simulink model "F16BlockASYM_JOY"  (R2012b)
settings: Solver=ode5  StartTime=0.0  StopTime=inf  FixedStep=0.02  RelTol=1e-3
InitFcn:
  | mex nlplantASYM.c
values from neighbouring files (symbols this model uses):
  DisEle_1 = ElevatorDis    (= 0)    [runF16Sim.m]
  DisEle_2 = -2*ElevatorDis    (= 0)    [runF16Sim.m]
  DisEle_3 = ElevatorDis    (= 0)    [runF16Sim.m]
  fi_flag_Simulink = 1    [runF16Sim.m]
  latitude = 52.073105    [runF16Sim.m]
  longitude = -000.616697    (= -0.616697)    [runF16Sim.m]
  Model_used_flag = 1    [runF16Sim.m]
undefined symbols (not defined in the file or in its folder): Earth, m, rad, s, trim_control, trim_state, trim_throttle, WGS84
libraries: F16_Actuator_Library x7, simulink x7, aerolibfltsims x3, aerolibtransform2 x2, aerolibconvert2 x2, aerolibatmos2 x2, aerolibasang x1, aerolibanimutils x1, aerolibconvert x1, aerolibobsolete x1, vrlib x1
settings Model: ExtModeAutoUpdateStatusClock=off  Creator=keviczky  LastModifiedBy=David
settings DataIOCC: Decimation=50  LimitDataPoints=off  SignalLoggingSaveFormat=ModelDataLogs  SignalLoggingName=sigsOut
settings OptimizationCC: BooleanDataType=off  InlineInvariantSignals=on
settings DebuggingCC: SaveWithParameterizedLinksMsg=none  SignalResolutionControl=TryResolveAllWithWarning  SolverPrmCheckMsg=none  MultiTaskDSMMsg=warning  MultiTaskCondExecSysMsg=none  StrictBusMsg=None
settings HardwareCC: TargetUnknown=on
settings RTWCC: IncludeERTFirstTime=on
settings GRTTargetCC: CombineOutputUpdateFcns=off  GRTInterface=on

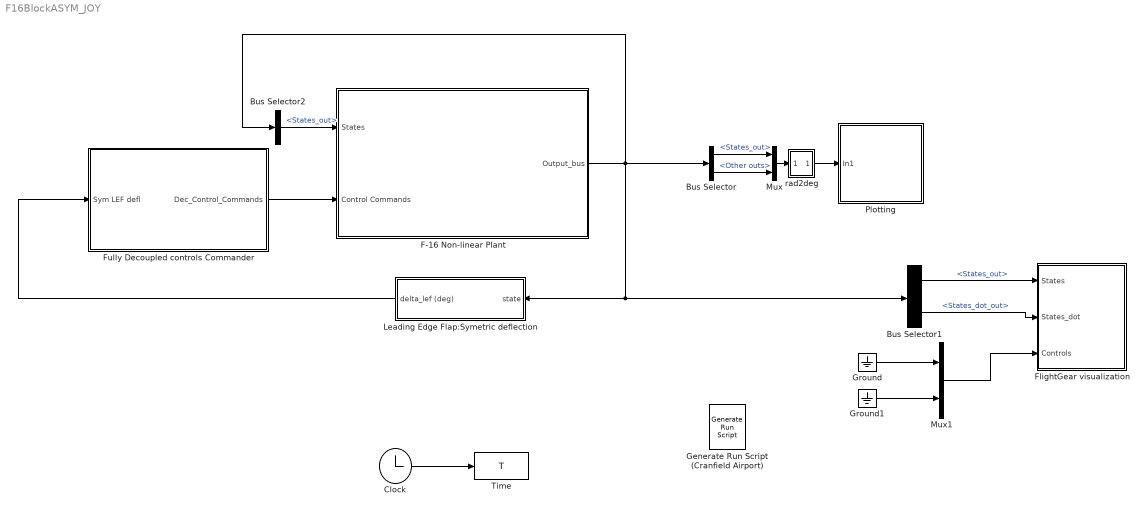
== system F16BlockASYM_JOY ==
  Bus Selector : BusSelector  OutputSignals=States_out,Other outs
  Bus Selector1 : BusSelector  OutputSignals=States_out,States_dot_out
  Bus Selector2 : BusSelector  OutputSignals=States_out
  Clock : Clock
      settings: Decimation=50
  F-16 Non-linear Plant : Subsystem
      mask Display:
      | image(imread('f16.jpg'))
      | port_label('output', 1, 'Out_bus')
      | port_label('input', 1, 'State_feedback')
      | port_label('input', 2, 'Control_Commands')
  FlightGear visualization : Subsystem  TreatAsAtomicUnit=on
  Fully Decoupled controls Commander : Subsystem
  Generate Run Script (Cranfield Airport) : aerolibfltsims/Generate Run Script  OutputFileName=runfg.bat  FlightGearBaseDirectory=C:\Program Files\FlightGear  GeometryModelName=f16  DestinationPort=5502  OriginAddress=127.0.0.1  OriginPort=5505  LocalAddress=127.0.0.1  AirportId=EGTC  RunwayId=1  InitialAltitude=trim_state(3)*3.2808399  InitialHeading=0  OffsetDistance=4.72  OffsetAzimuth=0  GenerateFile=off  Architecture=Win64  dataFlow=Send
  Ground : Ground
  Ground1 : Ground
  Leading Edge Flap:Symetric deflection : Subsystem
  Mux : Mux  Inputs=2
  Mux1 : Mux  Inputs=2
  Plotting : Subsystem
      mask Display: image(imread('f16output.jpg'))
  Time : ToWorkspace  VariableName=T  SampleTime=-1
      settings: Decimation=100
  rad2deg : Subsystem
  wires:
  Fully Decoupled controls Commander/1(Dec_Control_Commands) -> F-16 Non-linear Plant/2(Control Commands)
  Clock/1 -> Time/1
  rad2deg/1(Out1) -> Plotting/1(In1)
  Bus Selector/1 -> Mux/1  "<States_out>"
  Bus Selector/2 -> Mux/2  "<Other outs>"
  Mux/1 -> rad2deg/1(In1)
  F-16 Non-linear Plant/1(Output_bus) -> Bus Selector1/1, Leading Edge Flap:Symetric deflection/1(state), Bus Selector2/1, Bus Selector/1
  Bus Selector2/1 -> F-16 Non-linear Plant/1(States)  "<States_out>"
  Leading Edge Flap:Symetric deflection/1(delta_lef (deg)) -> Fully Decoupled controls Commander/1(Sym LEF defl)
  Ground/1 -> Mux1/1
  Ground1/1 -> Mux1/2
  Bus Selector1/1 -> FlightGear visualization/1(States)  "<States_out>"
  Bus Selector1/2 -> FlightGear visualization/2(States_dot)  "<States_dot_out>"
  Mux1/1 -> FlightGear visualization/3(Controls)

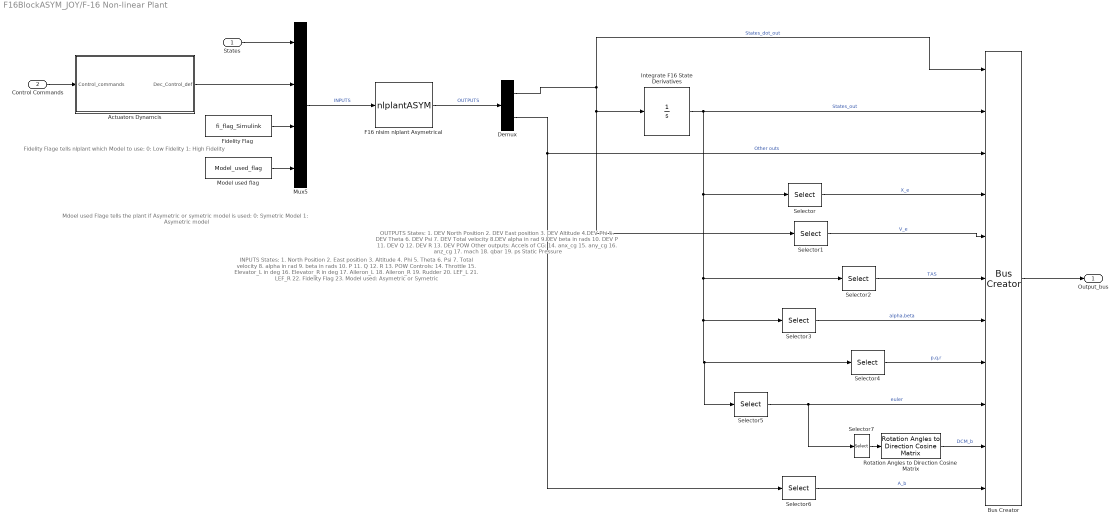
== system F16BlockASYM_JOY/F-16 Non-linear Plant ==
  note: OUTPUTS
      | States:
      | 1. DEV North Position
      | 2. DEV East position
      | 3. DEV Altitude
      | 4.DEV  Phi
      | 5. DEV Theta
      | 6. DEV Psi
      | 7. DEV Total velocity
      | 8.DEV alpha in rad
      | 9.DEV  beta in rads
      | 10. DEV P
      | 11. DEV Q
      | 12. DEV R
      | 13. DEV POW
      |
      | Other outputs:
      | Accels of CG:
      | 14. anx_cg
      | 15. any_cg
      | 16. anz_cg
      | 17. mach
      | 18. qbar
      | 19. ps   Static Pressure
  note: Fidelity Flage tells nlplant
      | which Model to use:
      | 0: Low Fidelity
      | 1: High Fidelity
  note: INPUTS
      | States:
      | 1. North Position
      | 2. East position
      | 3. Altitude
      | 4. Phi
      | 5. Theta
      | 6. Psi
      | 7. Total velocity
      | 8. alpha in rad
      | 9. beta in rads
      | 10. P
      | 11. Q
      | 12. R
      | 13. POW
      |
      | Controls:
      | 14. Throttle
      | 15. Elevator_L in deg
      | 16. Elevator_R in deg
      | 17. Aileron_L
      | 18. Aileron_R
      | 19. Rudder
      | 20. LEF_L
      | 21. LEF_R
      |
      | 22. Fidelity Flag
      |
      | 23. Model used: Asymetric or Symetric
  note: Mdoel used  Flage tells the plant
      |  if Asymetric or symetric model is used:
      | 0: Symetric Model
      | 1: Asymetric model
  States : Inport
  Control Commands : Inport  Port=2
  Actuators Dynamcis : Subsystem  TreatAsAtomicUnit=on
  Bus Creator : BusCreator  Inputs=11
  Demux : Demux  Outputs=[13 6]
  F16 nlsim nlplant Asymetrical : MATLABFcn  MATLABFcn=nlplantASYM  OutputDimensions=19  OutputSignalType=real
  Fidelity Flag : Constant  Value=fi_flag_Simulink
  Integrate F16 State Derivatives : Integrator  InitialCondition=trim_state
  Model used flag : Constant  Value=Model_used_flag
  Mux5 : Mux  Inputs=[13 8 1 1]
  Rotation Angles to Direction Cosine Matrix : aerolibtransform2/Rotation Angles to Direction Cosine Matrix  rotationOrder=ZYX
  Selector : Selector  InputPortWidth=13  IndexOptions=Index vector (dialog)  Indices=[1:3]  OutputSizes=1
  Selector1 : Selector  InputPortWidth=13  IndexOptions=Index vector (dialog)  Indices=[1:3]  OutputSizes=1
  Selector2 : Selector  InputPortWidth=13  IndexOptions=Index vector (dialog)  Indices=[7]  OutputSizes=1
  Selector3 : Selector  InputPortWidth=13  IndexOptions=Index vector (dialog)  Indices=[8:9]  OutputSizes=1
  Selector4 : Selector  InputPortWidth=13  IndexOptions=Index vector (dialog)  Indices=[10:12]  OutputSizes=1
  Selector5 : Selector  InputPortWidth=13  IndexOptions=Index vector (dialog)  Indices=[4:6]  OutputSizes=1
  Selector6 : Selector  InputPortWidth=6  IndexOptions=Index vector (dialog)  Indices=[1:3]  OutputSizes=1
  Selector7 : Selector  InputPortWidth=3  IndexOptions=Index vector (dialog)  Indices=[3 2 1]  OutputSizes=1
  Output_bus : Outport
  wires:
  Demux/1 -> Bus Creator/1, Selector1/1, Integrate F16 State Derivatives/1  "States_dot_out"
  Selector/1 -> Bus Creator/4  "X_e"
  Selector1/1 -> Bus Creator/5  "V_e"
  Selector2/1 -> Bus Creator/6  "TAS"
  Selector3/1 -> Bus Creator/7  "alpha,beta"
  Selector4/1 -> Bus Creator/8  "p,q,r"
  Selector5/1 -> Selector7/1, Bus Creator/9  "euler"
  Selector6/1 -> Bus Creator/11  "A_b"
  Demux/2 -> Selector6/1, Bus Creator/3  "Other outs"
  Selector7/1 -> Rotation Angles to Direction Cosine Matrix/1
  Integrate F16 State Derivatives/1 -> Selector5/1, Selector4/1, Selector3/1, Selector2/1, Selector/1, Bus Creator/2  "States_out"
  Rotation Angles to Direction Cosine Matrix/1 -> Bus Creator/10  "DCM_b"
  Bus Creator/1 -> Output_bus/1
  Fidelity Flag/1 -> Mux5/3
  Control Commands/1 -> Actuators Dynamcis/1(Control_commands)
  States/1 -> Mux5/1
  Mux5/1 -> F16 nlsim nlplant Asymetrical/1  "INPUTS"
  F16 nlsim nlplant Asymetrical/1 -> Demux/1  "OUTPUTS"
  Actuators Dynamcis/1(Dec_Control_def) -> Mux5/2
  Model used flag/1 -> Mux5/4

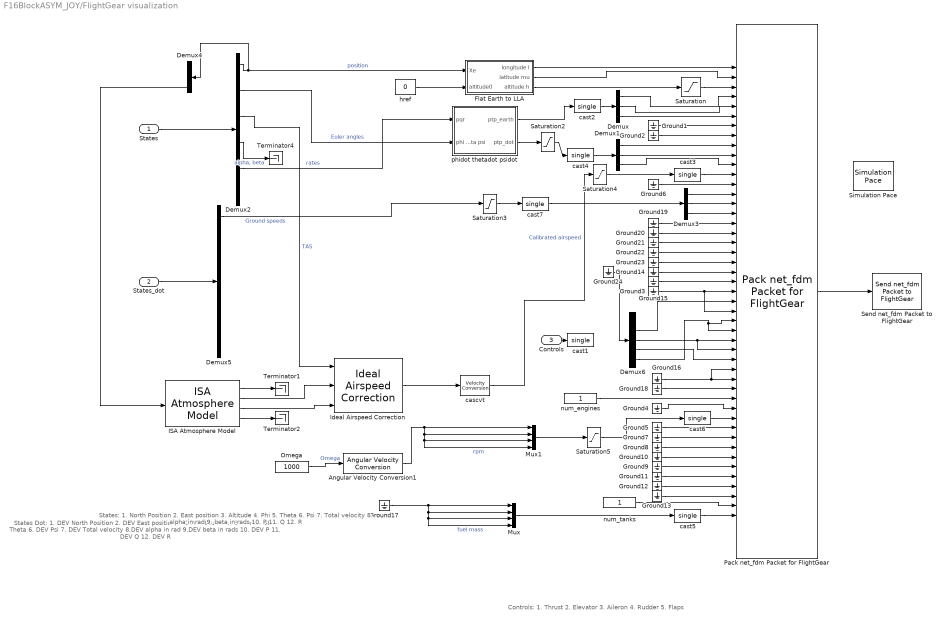
== system F16BlockASYM_JOY/FlightGear visualization ==
  note: States Dot:
      | 1. DEV North Position
      | 2. DEV East position
      | 3. DEV Altitude
      | 4.DEV  Phi
      | 5. DEV Theta
      | 6. DEV Psi
      | 7. DEV Total velocity
      | 8.DEV alpha in rad
      | 9.DEV  beta in rads
      | 10. DEV P
      | 11. DEV Q
      | 12. DEV R
  note: States:
      | 1. North Position
      | 2. East position
      | 3. Altitude
      | 4. Phi
      | 5. Theta
      | 6. Psi
      | 7. Total velocity
      | 8. alpha in rad
      | 9. beta in rads
      | 10. P
      | 11. Q
      | 12. R
  note: Controls:
      | 1. Thrust
      | 2. Elevator
      | 3. Aileron
      | 4. Rudder
      | 5. Flaps
  States : Inport
  States_dot : Inport  Port=2
  Controls : Inport  Port=3
  Angular Velocity Conversion1 : aerolibconvert2/Angular Velocity Conversion  IU=rad/s  OU=rpm
  Demux{,1,3..4} (4 alike) : Demux  Outputs=3
  Demux2 : Demux  Outputs=[3 3 1 2 3 1]
  Demux5 : Demux  Outputs=[3 3 1 2 3 1]
  Demux6 : Demux  Outputs=5
  Flat Earth to LLA : Subsystem
  Ground{1..24} (24 alike) : Ground
  ISA Atmosphere Model : aerolibatmos2/ISA Atmosphere Model  custom=off  g=9.80665  gamma=1.4  R=287.0531  L=0.0065  h_trop=11000  h_strat=20000  rho0=1.225  P0=101325  T0=288.15
  Ideal Airspeed Correction : aerolibasang/Ideal Airspeed Correction  units=Metric (MKS)  vel_in=TAS  vel_out_tas=CAS  vel_out_eas=CAS  vel_out_cas=TAS  action=Warning
  Mux : Mux
  Mux1 : Mux
  Omega : Constant  Value=1000  OutDataTypeStr=uint32
  Pack net_fdm Packet for FlightGear : aerolibfltsims/Pack net_fdm Packet for FlightGear  FlightGearVersion=v2.0  ShowPositionAttitudeInputs=on  ShowVelocityAccelerationInputs=on  ShowControlSurfacePositionInputs=on  ShowEngineFuelInputs=on  ShowLandingGearInputs=off  ShowEnvironmentInputs=off  SampleTime=-1
      settings: AttributesFormatString=FG VERSION: %<FlightGearVersion>
  Saturation : Saturate  UpperLimit=1e8  LowerLimit=-1e5
  Saturation2 : Saturate  UpperLimit=1e3  LowerLimit=-1e3
  Saturation3 : Saturate  UpperLimit=1e4  LowerLimit=-1e4
  Saturation4 : Saturate  UpperLimit=1e4  LowerLimit=-1e4
  Saturation5 : Saturate  UpperLimit=1e6  LowerLimit=0
  Send net_fdm Packet to FlightGear : aerolibfltsims/Send net_fdm Packet to FlightGear  DestinationIpAddress=127.0.0.1  DestinationPort=5502  LocalIpPort=-1  varLen=off  SampleTime=-1
  Simulation Pace : aerolibanimutils/Simulation Pace  SimulationPace=1  SleepMode=MATLAB Thread  OutputPaceError=off  SampleTime=.04
      settings: AttributesFormatString=%<SimulationPace> sec/sec
  Terminator1 : Terminator
  Terminator2 : Terminator
  Terminator4 : Terminator
  cascvt : aerolibconvert/Velocity Conversion  IU=m/s  OU=kts
  cast{1..7} (7 alike) : DataTypeConversion  OutDataTypeStr=single  SaturateOnIntegerOverflow=on
  href : Constant  Value=0  VectorParams1D=off
  num_engines : Constant  OutDataTypeStr=uint32
  num_tanks : Constant  OutDataTypeStr=uint32
  phidot thetadot psidot : Subsystem
  wires:
  Pack net_fdm Packet for FlightGear/1 -> Send net_fdm Packet to FlightGear/1
  Ground3/1 -> Pack net_fdm Packet for FlightGear/26, Pack net_fdm Packet for FlightGear/24
  Demux1/3 -> Pack net_fdm Packet for FlightGear/11
  Demux1/2 -> Pack net_fdm Packet for FlightGear/10
  Demux1/1 -> Pack net_fdm Packet for FlightGear/9
  Ground2/1 -> Pack net_fdm Packet for FlightGear/8
  Ground1/1 -> Pack net_fdm Packet for FlightGear/7
  Demux/3 -> Pack net_fdm Packet for FlightGear/6
  Demux/2 -> Pack net_fdm Packet for FlightGear/5
  Demux/1 -> Pack net_fdm Packet for FlightGear/4
  Ground6/1 -> Pack net_fdm Packet for FlightGear/13
  ISA Atmosphere Model/2 -> Ideal Airspeed Correction/2
  phidot thetadot psidot/2(ptp_dot) -> Saturation2/1
  phidot thetadot psidot/1(ptp_earth) -> cast2/1
  cast3/1 -> Pack net_fdm Packet for FlightGear/12
  Demux2/2 -> phidot thetadot psidot/2(phi theta psi)  "Euler angles"
  cascvt/1 -> Saturation4/1  "Calibrated airspeed"
  Ideal Airspeed Correction/1 -> cascvt/1
  Ground15/1 -> Pack net_fdm Packet for FlightGear/23
  Ground14/1 -> Pack net_fdm Packet for FlightGear/22
  Ground23/1 -> Pack net_fdm Packet for FlightGear/21
  Ground22/1 -> Pack net_fdm Packet for FlightGear/20
  Ground21/1 -> Pack net_fdm Packet for FlightGear/19
  Ground20/1 -> Pack net_fdm Packet for FlightGear/18
  Ground19/1 -> Pack net_fdm Packet for FlightGear/17
  href/1 -> Flat Earth to LLA/2(altitude0)
  Flat Earth to LLA/3(altitude h) -> Saturation/1
  States/1 -> Demux2/1
  Demux2/5 -> phidot thetadot psidot/1(pqr)  "rates"
  Flat Earth to LLA/1(longitude l) -> Pack net_fdm Packet for FlightGear/1
  Flat Earth to LLA/2(latitude mu) -> Pack net_fdm Packet for FlightGear/2
  Demux2/1 -> Flat Earth to LLA/1(Xe), Demux4/1  "position"
  Demux3/1 -> Pack net_fdm Packet for FlightGear/14
  Demux3/2 -> Pack net_fdm Packet for FlightGear/15
  Demux3/3 -> Pack net_fdm Packet for FlightGear/16
  Demux5/1 -> Saturation3/1  "Ground speeds"
  cast2/1 -> Demux/1
  cast4/1 -> Demux1/1
  Demux2/4 -> Terminator4/1  "alpha, beta"
  cast5/1 -> Pack net_fdm Packet for FlightGear/47
  cast6/1 -> Pack net_fdm Packet for FlightGear/37
  num_tanks/1 -> Pack net_fdm Packet for FlightGear/46
  Demux2/3 -> Ideal Airspeed Correction/1  "TAS"
  ISA Atmosphere Model/1 -> Terminator1/1
  ISA Atmosphere Model/4 -> Terminator2/1
  ISA Atmosphere Model/3 -> Ideal Airspeed Correction/3
  Demux4/3 -> ISA Atmosphere Model/1
  Ground17/1 -> Mux/2, Mux/3, Mux/4, Mux/1  "fuel mass"
  Mux/1 -> cast5/1
  Omega/1 -> Angular Velocity Conversion1/1  "Omega"
  Mux1/1 -> Saturation5/1
  cast7/1 -> Demux3/1
  Angular Velocity Conversion1/1 -> Mux1/2, Mux1/3, Mux1/4, Mux1/1  "rpm"
  Saturation/1 -> Pack net_fdm Packet for FlightGear/3
  Saturation2/1 -> cast4/1
  Saturation3/1 -> cast7/1
  Saturation4/1 -> cast3/1
  Saturation5/1 -> cast6/1
  States_dot/1 -> Demux5/1
  Ground5/1 -> Pack net_fdm Packet for FlightGear/38
  Ground7/1 -> Pack net_fdm Packet for FlightGear/39
  Ground8/1 -> Pack net_fdm Packet for FlightGear/40
  Ground10/1 -> Pack net_fdm Packet for FlightGear/41
  Ground9/1 -> Pack net_fdm Packet for FlightGear/42
  Ground11/1 -> Pack net_fdm Packet for FlightGear/43
  Ground12/1 -> Pack net_fdm Packet for FlightGear/44
  Ground13/1 -> Pack net_fdm Packet for FlightGear/45
  Ground4/1 -> Pack net_fdm Packet for FlightGear/36
  num_engines/1 -> Pack net_fdm Packet for FlightGear/35
  Controls/1 -> cast1/1
  Demux6/3 -> Pack net_fdm Packet for FlightGear/29, Pack net_fdm Packet for FlightGear/30
  Demux6/4 -> Pack net_fdm Packet for FlightGear/31
  Demux6/5 -> Pack net_fdm Packet for FlightGear/27, Pack net_fdm Packet for FlightGear/28
  Ground18/1 -> Pack net_fdm Packet for FlightGear/34
  Ground16/1 -> Pack net_fdm Packet for FlightGear/32, Pack net_fdm Packet for FlightGear/33
  Demux6/2 -> Pack net_fdm Packet for FlightGear/25
  Ground24/1 -> Demux6/1

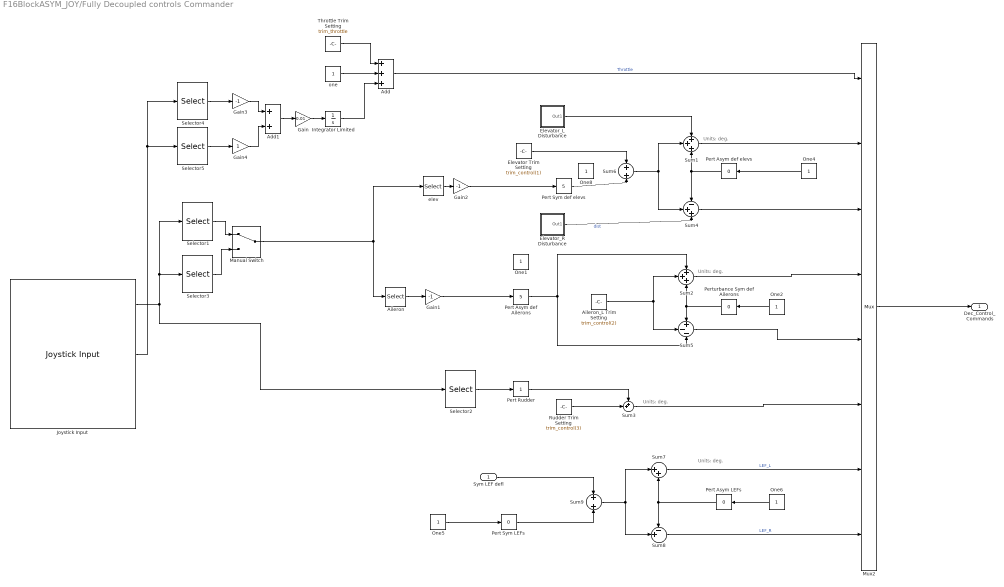
== system F16BlockASYM_JOY/Fully Decoupled controls Commander ==
  note: Units: deg.
  note: Units: deg.
  note: Units: deg.
  note: Units: deg.
  Sym LEF defl : Inport
  Add : Sum  Inputs=+++
  Add1 : Sum
  Aileron : Selector  InputPortWidth=2  IndexOptions=Index vector (dialog)  Indices=1  OutputSizes=1
  Aileron_L Trim Setting : Constant  Value=trim_control(2)
  Elevator Trim Setting : Constant  Value=trim_control(1)  VectorParams1D=off
  Elevator_L Disturbance : Subsystem
  Elevator_R Disturbance : Subsystem
  Gain : Gain  Gain=0.01
  Gain1 : Gain  Gain=-1
  Gain2 : Gain  Gain=-1
  Gain3 : Gain  Gain=-1
  Gain4 : Gain
  Integrator Limited : Integrator  LimitOutput=on  UpperSaturationLimit=350  LowerSaturationLimit=0
  Joystick Input : vrlib/Joystick Input  joyid=1  adjustports=on  forcefeed=off
  Manual Switch : ManualSwitch
  Mux2 : Mux  Inputs=8
  One{1..2,4..6,8} (6 alike) : Constant
  Pert Asym LEFs : simulink/Math Operations/Slider Gain  low=-50  gain=0  high=50
  Pert Asym def Ailerons : simulink/Math Operations/Slider Gain  low=-50  gain=5  high=50
  Pert Asym def elevs : simulink/Math Operations/Slider Gain  low=-50  gain=0  high=50
  Pert Rudder : simulink/Math Operations/Slider Gain  low=-50  gain=1  high=50
  Pert Sym LEFs : simulink/Math Operations/Slider Gain  low=-50  gain=0  high=50
  Pert Sym def elevs : simulink/Math Operations/Slider Gain  low=-50  gain=5  high=50
  Perturbance Sym def Ailerons : simulink/Math Operations/Slider Gain  low=-50  gain=0  high=50
  Rudder Trim Setting : Constant  Value=trim_control(3)
  Selector1 : Selector  InputPortWidth=5  IndexOptions=Index vector (dialog)  Indices=1:2  OutputSizes=1
  Selector2 : Selector  InputPortWidth=5  IndexOptions=Index vector (dialog)  Indices=3  OutputSizes=1
  Selector3 : Selector  InputPortWidth=5  IndexOptions=Index vector (dialog)  Indices=4:5  OutputSizes=1
  Selector4 : Selector  InputPortWidth=10  IndexOptions=Index vector (dialog)  Indices=1  OutputSizes=1
  Selector5 : Selector  InputPortWidth=10  IndexOptions=Index vector (dialog)  Indices=4  OutputSizes=1
  Sum1 : Sum  Inputs=+++  SaturateOnIntegerOverflow=on  InputSameDT=on  OutDataTypeStr=Inherit: Same as first input
  Sum2 : Sum  Inputs=+++  SaturateOnIntegerOverflow=on  InputSameDT=on  OutDataTypeStr=Inherit: Same as first input
  Sum3 : Sum  Inputs=++|  SaturateOnIntegerOverflow=on  InputSameDT=on  OutDataTypeStr=Inherit: Same as first input
  Sum4 : Sum  Inputs=-++  SaturateOnIntegerOverflow=on  InputSameDT=on  OutDataTypeStr=Inherit: Same as first input
  Sum5 : Sum  Inputs=+--  SaturateOnIntegerOverflow=on  InputSameDT=on  OutDataTypeStr=Inherit: Same as first input
  Sum6 : Sum  SaturateOnIntegerOverflow=on  InputSameDT=on  OutDataTypeStr=Inherit: Same as first input
  Sum7 : Sum  Inputs=|++  SaturateOnIntegerOverflow=on  InputSameDT=on  OutDataTypeStr=Inherit: Same as first input
  Sum8 : Sum  Inputs=-+|  SaturateOnIntegerOverflow=on  InputSameDT=on  OutDataTypeStr=Inherit: Same as first input
  Sum9 : Sum  SaturateOnIntegerOverflow=on  InputSameDT=on  OutDataTypeStr=Inherit: Same as first input
  Throttle Trim Setting : Constant  Value=trim_throttle
  elev : Selector  InputPortWidth=2  IndexOptions=Index vector (dialog)  Indices=2  OutputSizes=1
  one : Constant
  Dec_Control_Commands : Outport
  wires:
  Add/1 -> Mux2/1  "Throttle"
  Mux2/1 -> Dec_Control_Commands/1
  Sum2/1 -> Mux2/4
  Sum3/1 -> Mux2/6
  Pert Rudder/1 -> Sum3/1
  Rudder Trim Setting/1 -> Sum3/2
  Pert Asym def Ailerons/1 -> Sum5/3, Sum2/1
  Sum5/1 -> Mux2/5
  One2/1 -> Perturbance Sym def Ailerons/1
  Perturbance Sym def Ailerons/1 -> Sum5/1, Sum2/3
  Aileron_L Trim Setting/1 -> Sum2/2, Sum5/2
  Sum1/1 -> Mux2/2
  Elevator_L Disturbance/1(Out1) -> Sum1/1
  Sum4/1 -> Mux2/3
  elev/1 -> Gain2/1
  Elevator_R Disturbance/1(Out1) -> Sum4/3  "dist"
  Pert Sym def elevs/1 -> Sum6/2
  Elevator Trim Setting/1 -> Sum6/1
  Sum6/1 -> Sum4/2, Sum1/2
  One4/1 -> Pert Asym def elevs/1
  Pert Asym def elevs/1 -> Sum4/1, Sum1/3
  Sum7/1 -> Mux2/7  "LEF_L"
  Sum8/1 -> Mux2/8  "LEF_R"
  One5/1 -> Pert Sym LEFs/1
  Pert Sym LEFs/1 -> Sum9/2
  Sym LEF defl/1 -> Sum9/1
  Sum9/1 -> Sum8/2, Sum7/1
  One6/1 -> Pert Asym LEFs/1
  Pert Asym LEFs/1 -> Sum8/1, Sum7/2
  Aileron/1 -> Gain1/1
  Selector2/1 -> Pert Rudder/1
  Manual Switch/1 -> Aileron/1, elev/1
  one/1 -> Add/2
  Gain2/1 -> Pert Sym def elevs/1
  Gain1/1 -> Pert Asym def Ailerons/1
  Integrator Limited/1 -> Add/3
  Throttle Trim Setting/1 -> Add/1
  Joystick Input/1 -> Selector3/1, Selector1/1, Selector2/1
  Selector1/1 -> Manual Switch/1
  Selector3/1 -> Manual Switch/2
  Joystick Input/2 -> Selector5/1, Selector4/1
  Selector4/1 -> Gain3/1
  Selector5/1 -> Gain4/1
  Gain3/1 -> Add1/1
  Gain4/1 -> Add1/2
  Add1/1 -> Gain/1
  Gain/1 -> Integrator Limited/1

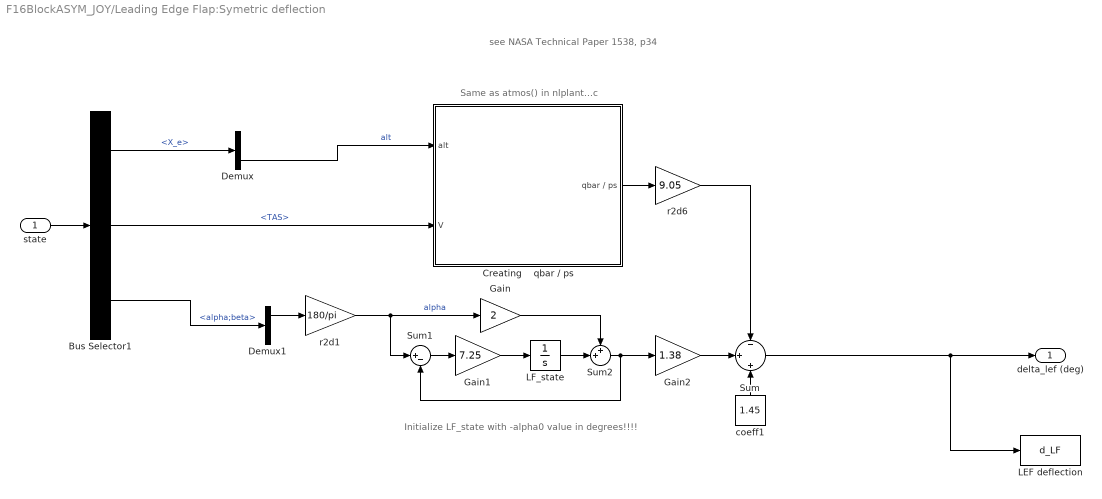
== system F16BlockASYM_JOY/Leading Edge Flap:Symetric deflection ==
  note: see NASA Technical Paper 1538, p34
  note: Same as atmos() in nlplant...c
  note: Initialize LF_state with -alpha0 value in degrees!!!!
  state : Inport
  Bus Selector1 : BusSelector  OutputSignals=X_e,TAS,alpha;beta
  Creating    qbar / ps : Subsystem
  Demux : Demux  Outputs=3
  Demux1 : Demux  Outputs=2
  Gain : Gain  Gain=2  SaturateOnIntegerOverflow=on  OutDataTypeStr=Inherit: Same as input  ParamDataTypeStr=Inherit: Same as input
  Gain1 : Gain  Gain=7.25  SaturateOnIntegerOverflow=on  OutDataTypeStr=Inherit: Same as input  ParamDataTypeStr=Inherit: Same as input
  Gain2 : Gain  Gain=1.38  SaturateOnIntegerOverflow=on  OutDataTypeStr=Inherit: Same as input  ParamDataTypeStr=Inherit: Same as input
  LEF deflection : ToWorkspace  VariableName=d_LF  SampleTime=-1
      settings: Decimation=100
  LF_state : Integrator  InitialCondition=-trim_state(8)*180/pi
  Sum : Sum  Inputs=-|+|+  SaturateOnIntegerOverflow=on  InputSameDT=on  OutDataTypeStr=Inherit: Same as first input
  Sum1 : Sum  Inputs=|+-  SaturateOnIntegerOverflow=on  InputSameDT=on  OutDataTypeStr=Inherit: Same as first input
  Sum2 : Sum  Inputs=++|  SaturateOnIntegerOverflow=on  InputSameDT=on  OutDataTypeStr=Inherit: Same as first input
  coeff1 : Constant  Value=1.45
  r2d1 : Gain  Gain=180/pi  SaturateOnIntegerOverflow=on  OutDataTypeStr=Inherit: Same as input  ParamDataTypeStr=Inherit: Same as input
  r2d6 : Gain  Gain=9.05  SaturateOnIntegerOverflow=on  OutDataTypeStr=Inherit: Same as input  ParamDataTypeStr=Inherit: Same as input
  delta_lef (deg) : Outport
  wires:
  Sum/1 -> LEF deflection/1, delta_lef (deg)/1
  state/1 -> Bus Selector1/1
  Sum1/1 -> Gain1/1
  Gain1/1 -> LF_state/1
  Gain/1 -> Sum2/1
  Gain2/1 -> Sum/2
  Demux1/1 -> r2d1/1
  coeff1/1 -> Sum/3
  Sum2/1 -> Sum1/2, Gain2/1
  LF_state/1 -> Sum2/2
  r2d1/1 -> Sum1/1, Gain/1  "alpha"
  Bus Selector1/2 -> Creating    qbar / ps/2(V)  "<TAS>"
  Creating    qbar / ps/1(qbar / ps) -> r2d6/1
  r2d6/1 -> Sum/1
  Demux/3 -> Creating    qbar / ps/1(alt)  "alt"
  Bus Selector1/1 -> Demux/1  "<X_e>"
  Bus Selector1/3 -> Demux1/1  "<alpha;beta>"

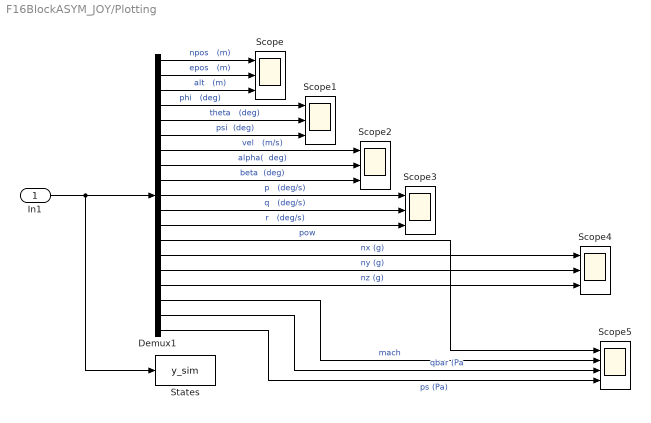
== system F16BlockASYM_JOY/Plotting ==
  In1 : Inport
  Demux1 : Demux  Outputs=19
  Scope{,1..4} (5 alike) : Scope  NumInputPorts=3
      Scope settings: YMin=12100~6e-11~13235  YMax=13700~8.75e-11~13320  Decimation=20
      Scope1 settings: TimeRange=10  YMin=-0.5~2.5~0  YMax=8~22.5~12  Decimation=20
      Scope2 settings: YMin=101~22.15~1.19  YMax=104.5~22.215~1.39  SaveName=ScopeData2  Decimation=20
      Scope3 settings: YMin=-5~-5~-5  YMax=5~5~5  SaveName=ScopeData3  Decimation=20
      Scope4 settings: YMin=-5~-5~-5  YMax=5~5~5  SaveName=ScopeData4  Decimation=20
  Scope5 : Scope  NumInputPorts=4
      settings: YMin=-5~-5~-5~-5  YMax=5~5~5~5  SaveName=ScopeData5  Decimation=20
  States : ToWorkspace  VariableName=y_sim  SampleTime=-1
      settings: Decimation=100
  wires:
  Demux1/1 -> Scope/1  "npos   (m)"
  Demux1/2 -> Scope/2  "epos   (m)"
  Demux1/3 -> Scope/3  "alt   (m)"
  Demux1/5 -> Scope1/2  "theta   (deg)"
  Demux1/6 -> Scope1/3  "psi  (deg)"
  Demux1/7 -> Scope2/1  "vel   (m/s)"
  Demux1/8 -> Scope2/2  "alpha(  deg)"
  Demux1/9 -> Scope2/3  "beta  (deg)"
  Demux1/10 -> Scope3/1  "p   (deg/s)"
  Demux1/11 -> Scope3/2  "q   (deg/s)"
  Demux1/12 -> Scope3/3  "r   (deg/s)"
  Demux1/14 -> Scope4/1  "nx (g)"
  Demux1/15 -> Scope4/2  "ny (g)"
  Demux1/16 -> Scope4/3  "nz (g)"
  Demux1/4 -> Scope1/1  "phi   (deg)"
  Demux1/17 -> Scope5/2  "mach"
  Demux1/18 -> Scope5/3  "qbar (Pa"
  Demux1/19 -> Scope5/4  "ps (Pa)"
  In1/1 -> Demux1/1, States/1
  Demux1/13 -> Scope5/1  "pow"

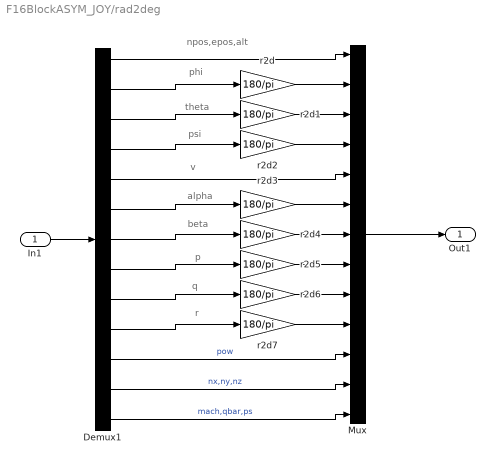
== system F16BlockASYM_JOY/rad2deg ==
  note: npos,epos,alt
  note: phi
  note: theta
  note: psi
  note: v
  note: alpha
  note: beta
  note: p
  note: q
  note: r
  In1 : Inport
  Demux1 : Demux  Outputs=[3 1 1 1 1 1 1 1 1 1 1 3 3]
  Mux : Mux  Inputs=[3 1 1 1 1 1 1 1 1 1 1 3 3]
  r2d{,1..7} (8 alike) : Gain  Gain=180/pi  SaturateOnIntegerOverflow=on  OutDataTypeStr=Inherit: Same as input  ParamDataTypeStr=Inherit: Same as input
  Out1 : Outport
  wires:
  In1/1 -> Demux1/1
  Demux1/2 -> r2d/1
  Demux1/3 -> r2d1/1
  Demux1/4 -> r2d2/1
  Demux1/1 -> Mux/1
  Demux1/5 -> Mux/5
  r2d2/1 -> Mux/4
  r2d1/1 -> Mux/3
  r2d/1 -> Mux/2
  Demux1/6 -> r2d3/1
  Demux1/7 -> r2d4/1
  Demux1/8 -> r2d5/1
  Demux1/9 -> r2d6/1
  Demux1/10 -> r2d7/1
  r2d4/1 -> Mux/7
  r2d5/1 -> Mux/8
  r2d6/1 -> Mux/9
  r2d7/1 -> Mux/10
  Mux/1 -> Out1/1
  Demux1/12 -> Mux/12  "nx,ny,nz"
  Demux1/13 -> Mux/13  "mach,qbar,ps"
  r2d3/1 -> Mux/6
  Demux1/11 -> Mux/11  "pow"

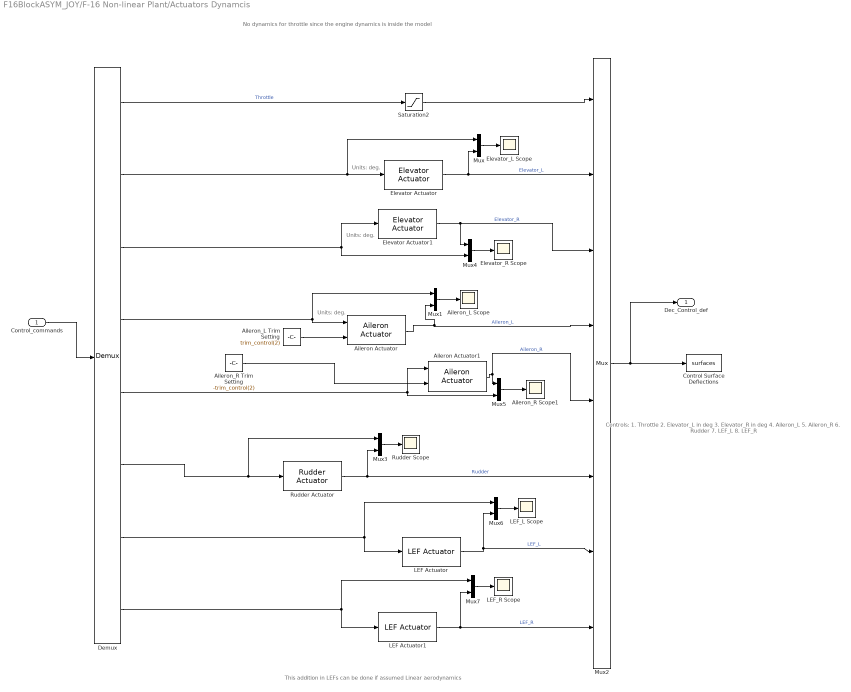
== system F16BlockASYM_JOY/F-16 Non-linear Plant/Actuators Dynamcis ==
  note: No dynamics for throttle since the engine dynamics is inside the model
  note: This addition in LEFs can be done
      |  if assumed Linear aerodynamics
  note: Units: deg.
  note: Units: deg.
  note: Units: deg.
  note: Controls:
      | 1. Throttle
      | 2. Elevator_L in deg
      | 3. Elevator_R in deg
      | 4. Aileron_L
      | 5. Aileron_R
      | 6. Rudder
      | 7. LEF_L
      | 8. LEF_R
  Control_commands : Inport
  Aileron Actuator : F16_Actuator_Library/Aileron Actuator
  Aileron Actuator1 : F16_Actuator_Library/Aileron Actuator
  Aileron_L Scope : Scope
      settings: TimeRange=30  SaveName=ScopeData7
  Aileron_L Trim Setting : Constant  Value=trim_control(2)
  Aileron_R Scope1 : Scope
      settings: TimeRange=30  SaveName=ScopeData10
  Aileron_R Trim Setting : Constant  Value=-trim_control(2)
  Control Surface Deflections : ToWorkspace  VariableName=surfaces  SampleTime=-1
      settings: Decimation=100
  Demux : Demux  Outputs=8
  Elevator Actuator : F16_Actuator_Library/Elevator Actuator
  Elevator Actuator1 : F16_Actuator_Library/Elevator Actuator
  Elevator_L Scope : Scope
      settings: TimeRange=5  YMin=-2.58372  YMax=-2.33766  SaveName=ScopeData6
  Elevator_R Scope : Scope
      settings: TimeRange=5  YMin=-2.58372  YMax=-2.33766  SaveName=ScopeData9
  LEF Actuator : F16_Actuator_Library/LEF Actuator
  LEF Actuator1 : F16_Actuator_Library/LEF Actuator
  LEF_L Scope : Scope
      settings: SaveName=ScopeData11
  LEF_R Scope : Scope
      settings: SaveName=ScopeData12
  Mux{,1,3..7} (7 alike) : Mux  Inputs=2
  Mux2 : Mux  Inputs=8
  Rudder Actuator : F16_Actuator_Library/Rudder Actuator
  Rudder Scope : Scope
      settings: SaveName=ScopeData8
  Saturation2 : Saturate  UpperLimit=1  LowerLimit=0
  Dec_Control_def : Outport
  wires:
  Control_commands/1 -> Demux/1
  Demux/1 -> Saturation2/1  "Throttle"
  Demux/2 -> Mux/1, Elevator Actuator/1
  Mux2/1 -> Dec_Control_def/1, Control Surface Deflections/1
  Elevator Actuator/1 -> Mux/2, Mux2/2  "Elevator_L"
  Mux/1 -> Elevator_L Scope/1
  Demux/4 -> Mux1/1, Aileron Actuator/1
  Demux/6 -> Rudder Actuator/1, Mux3/1
  Aileron Actuator/1 -> Mux1/2, Mux2/4  "Aileron_L"
  Rudder Actuator/1 -> Mux3/2, Mux2/6  "Rudder"
  Mux1/1 -> Aileron_L Scope/1
  Mux3/1 -> Rudder Scope/1
  Demux/3 -> Elevator Actuator1/1, Mux4/2
  Elevator Actuator1/1 -> Mux4/1, Mux2/3  "Elevator_R"
  Mux4/1 -> Elevator_R Scope/1
  Demux/5 -> Mux5/2, Aileron Actuator1/1
  Aileron Actuator1/1 -> Mux5/1, Mux2/5  "Aileron_R"
  Mux5/1 -> Aileron_R Scope1/1
  Demux/7 -> LEF Actuator/1, Mux6/1
  LEF Actuator/1 -> Mux6/2, Mux2/7  "LEF_L"
  Mux6/1 -> LEF_L Scope/1
  Demux/8 -> LEF Actuator1/1, Mux7/1
  LEF Actuator1/1 -> Mux2/8, Mux7/2  "LEF_R"
  Mux7/1 -> LEF_R Scope/1
  Aileron_L Trim Setting/1 -> Aileron Actuator/2
  Aileron_R Trim Setting/1 -> Aileron Actuator1/2
  Saturation2/1 -> Mux2/1

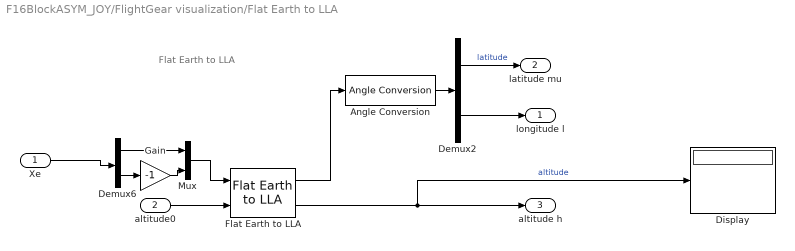
== system F16BlockASYM_JOY/FlightGear visualization/Flat Earth to LLA ==
  note: Flat Earth to LLA
  Xe : Inport
  altitude0 : Inport  Port=2
  Angle Conversion : aerolibconvert2/Angle Conversion  IU=deg  OU=rad
  Demux2 : Demux  Outputs=2
  Demux6 : Demux  Outputs=[2 1]
  Display : Display
  Flat Earth to LLA : aerolibtransform2/Flat Earth to LLA  units=Metric (MKS)  ptype=Earth (WGS84)  F=1/298.257223563  R=6378137  LL0=[latitude longitude]  psi=0
  Gain : Gain  Gain=-1
  Mux : Mux  Inputs=2
  longitude l : Outport
  latitude mu : Outport  Port=2
  altitude h : Outport  Port=3
  wires:
  Flat Earth to LLA/1 -> Angle Conversion/1
  Demux2/1 -> latitude mu/1  "latitude"
  Demux2/2 -> longitude l/1
  Xe/1 -> Demux6/1
  altitude0/1 -> Flat Earth to LLA/2
  Flat Earth to LLA/2 -> Display/1, altitude h/1  "altitude"
  Angle Conversion/1 -> Demux2/1
  Mux/1 -> Flat Earth to LLA/1
  Demux6/1 -> Mux/1
  Demux6/2 -> Gain/1
  Gain/1 -> Mux/2

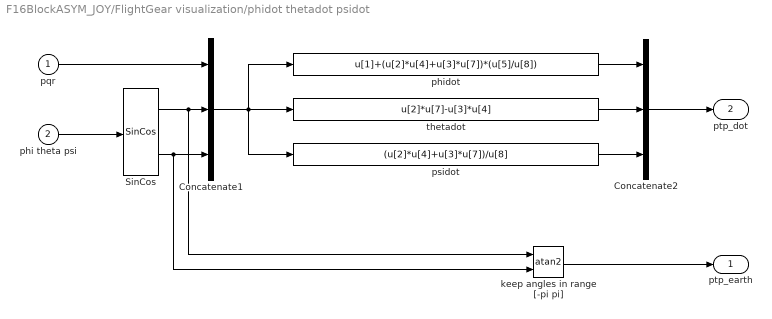
== system F16BlockASYM_JOY/FlightGear visualization/phidot thetadot psidot ==
  pqr : Inport
  phi theta psi : Inport  Port=2
  Concatenate1 : Concatenate  NumInputs=3
  Concatenate2 : Concatenate  NumInputs=3
  SinCos : aerolibobsolete/SinCos
  keep angles in range [-pi pi] : Trigonometry  Operator=atan2
  phidot : Fcn  Expr=u[1]+(u[2]*u[4]+u[3]*u[7])*(u[5]/u[8])
  psidot : Fcn  Expr=(u[2]*u[4]+u[3]*u[7])/u[8]
  thetadot : Fcn  Expr=u[2]*u[7]-u[3]*u[4]
  ptp_earth : Outport
  ptp_dot : Outport  Port=2
  wires:
  SinCos/2 -> Concatenate1/3, keep angles in range [-pi pi]/2
  SinCos/1 -> Concatenate1/2, keep angles in range [-pi pi]/1
  Concatenate2/1 -> ptp_dot/1
  phidot/1 -> Concatenate2/1
  thetadot/1 -> Concatenate2/2
  psidot/1 -> Concatenate2/3
  phi theta psi/1 -> SinCos/1
  pqr/1 -> Concatenate1/1
  Concatenate1/1 -> thetadot/1, phidot/1, psidot/1
  keep angles in range [-pi pi]/1 -> ptp_earth/1

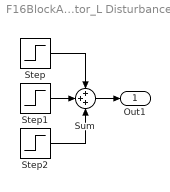
== system F16BlockASYM_JOY/Fully Decoupled controls Commander/Elevator_L Disturbance ==
  Step : Step  After=DisEle_1  SampleTime=0
  Step1 : Step  Time=3  After=DisEle_2  SampleTime=0
  Step2 : Step  Time=5  After=DisEle_3  SampleTime=0
  Sum : Sum  Inputs=+++  SaturateOnIntegerOverflow=on  InputSameDT=on  OutDataTypeStr=Inherit: Same as first input
  Out1 : Outport
  wires:
  Step1/1 -> Sum/2
  Step/1 -> Sum/1
  Step2/1 -> Sum/3
  Sum/1 -> Out1/1

== system F16BlockASYM_JOY/Fully Decoupled controls Commander/Elevator_R Disturbance ==
  Step : Step  After=DisEle_1  SampleTime=0
  Step1 : Step  Time=3  After=DisEle_2  SampleTime=0
  Step2 : Step  Time=5  After=DisEle_3  SampleTime=0
  Sum : Sum  Inputs=+++  SaturateOnIntegerOverflow=on  InputSameDT=on  OutDataTypeStr=Inherit: Same as first input
  Out1 : Outport
  wires:
  Step1/1 -> Sum/2
  Step/1 -> Sum/1
  Step2/1 -> Sum/3
  Sum/1 -> Out1/1

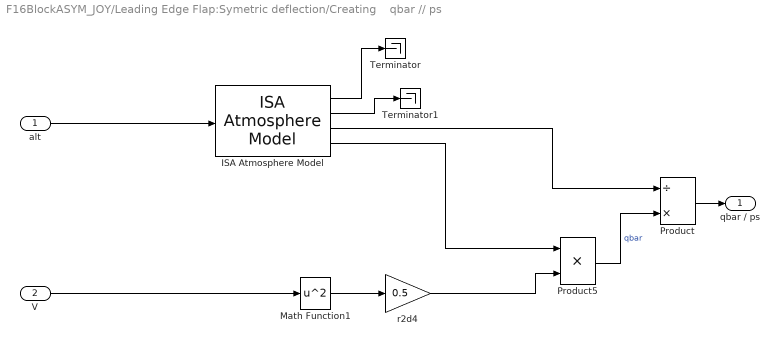
== system F16BlockASYM_JOY/Leading Edge Flap:Symetric deflection/Creating    qbar // ps ==
  alt : Inport
  V : Inport  Port=2
  ISA Atmosphere Model : aerolibatmos2/ISA Atmosphere Model  custom=off  g=9.80665  gamma=1.4  R=287.0531  L=0.0065  h_trop=11000  h_strat=20000  rho0=1.225  P0=101325  T0=288.15
  Math Function1 : Math  Operator=square  SaturateOnIntegerOverflow=on
  Product : Product  Inputs=/*  SaturateOnIntegerOverflow=on  InputSameDT=on  OutDataTypeStr=Inherit: Same as first input
  Product5 : Product  Inputs=**  SaturateOnIntegerOverflow=on  InputSameDT=on  OutDataTypeStr=Inherit: Same as first input
  Terminator : Terminator
  Terminator1 : Terminator
  r2d4 : Gain  Gain=0.5  SaturateOnIntegerOverflow=on  OutDataTypeStr=Inherit: Same as input  ParamDataTypeStr=Inherit: Same as input
  qbar / ps : Outport
  wires:
  alt/1 -> ISA Atmosphere Model/1
  Math Function1/1 -> r2d4/1
  r2d4/1 -> Product5/2
  Product5/1 -> Product/2  "qbar"
  V/1 -> Math Function1/1
  Product/1 -> qbar / ps/1
  ISA Atmosphere Model/4 -> Product5/1
  ISA Atmosphere Model/3 -> Product/1
  ISA Atmosphere Model/1 -> Terminator/1
  ISA Atmosphere Model/2 -> Terminator1/1
